simulink model "Demo_DSRC_DNPW_cs"  (Simulink 7.6)
settings: Solver=ode5  SolverMode=SingleTasking  StartTime=0.0  StopTime=5  FixedStep=1/20  RelTol=1e-3
PreLoadFcn:
  | check_NUTS_defined;
  | 
  | assignin('base',['model_closed_' bdroot],false);
InitFcn:
  | PreScanExperimentInitFcn(bdroot)
StopFcn:
  | PreScanExperimentStopFcn(bdroot)
undefined symbols (not defined in the file): DiscIntNeverNeededParam, spare_1, spare_10, spare_11, spare_12, spare_13, spare_14, spare_15, spare_16, spare_17, spare_18, spare_19, spare_2, spare_3, spare_4, spare_5, spare_6, spare_7, spare_8, spare_9
libraries: PreScanSimulinkLibrary x29, PreScanUsefulBlocks x11, simulink x9, simulink_extras x2
(part 3 of 6)

== system Demo_DSRC_DNPW_cs/STATE_HMI_Warning_Left ==
  State : Inport  SampleTime=TimeStep
  Acceleration : Subsystem  mask(ToSensorWorld){PortName=Acceleration_HMI_Warning_Left, PortIndex=212, PortWidth=3, TimeStep=1/20}
      mask prompts: PortName "Port Name [-]"; PortIndex "Index [-]"; PortWidth "Port Dimensions [-]"; TimeStep "Upload Period [s]"
      mask help: Sends signal(s) from Simulink to the Sensor World
      mask Help:
      | Sends signal(s) from Simulink to the Sensor World.
      | 
      | - Port Name [-]: specifies the name of the output terminal of the Simulink block.
      | - Index [-]: specifies the start position in the output vector sent to the Sensor World
      | - Port dimensions [-]: specifies the width (number of scalars) of the output port
      | - Upload period [s]: specifies the upload period (in seconds) of the port.
      mask Display: port_label('input', 1, PortName)
  Demux : Demux  Outputs=5
  Position : Subsystem  mask(ToSensorWorld){PortName=Position_HMI_Warning_Left, PortIndex=206, PortWidth=3, TimeStep=1/20}
      mask prompts: PortName "Port Name [-]"; PortIndex "Index [-]"; PortWidth "Port Dimensions [-]"; TimeStep "Upload Period [s]"
      mask help: Sends signal(s) from Simulink to the Sensor World
      mask Help:
      | Sends signal(s) from Simulink to the Sensor World.
      | 
      | - Port Name [-]: specifies the name of the output terminal of the Simulink block.
      | - Index [-]: specifies the start position in the output vector sent to the Sensor World
      | - Port dimensions [-]: specifies the width (number of scalars) of the output port
      | - Upload period [s]: specifies the upload period (in seconds) of the port.
      mask Display: port_label('input', 1, PortName)
  RPY : Subsystem  mask(ToSensorWorld){PortName=RPY_HMI_Warning_Left, PortIndex=215, PortWidth=3, TimeStep=1/20}
      mask prompts: PortName "Port Name [-]"; PortIndex "Index [-]"; PortWidth "Port Dimensions [-]"; TimeStep "Upload Period [s]"
      mask help: Sends signal(s) from Simulink to the Sensor World
      mask Help:
      | Sends signal(s) from Simulink to the Sensor World.
      | 
      | - Port Name [-]: specifies the name of the output terminal of the Simulink block.
      | - Index [-]: specifies the start position in the output vector sent to the Sensor World
      | - Port dimensions [-]: specifies the width (number of scalars) of the output port
      | - Upload period [s]: specifies the upload period (in seconds) of the port.
      mask Display: port_label('input', 1, PortName)
  Velocity : Subsystem  mask(ToSensorWorld){PortName=Velocity_HMI_Warning_Left, PortIndex=209, PortWidth=3, TimeStep=1/20}
      mask prompts: PortName "Port Name [-]"; PortIndex "Index [-]"; PortWidth "Port Dimensions [-]"; TimeStep "Upload Period [s]"
      mask help: Sends signal(s) from Simulink to the Sensor World
      mask Help:
      | Sends signal(s) from Simulink to the Sensor World.
      | 
      | - Port Name [-]: specifies the name of the output terminal of the Simulink block.
      | - Index [-]: specifies the start position in the output vector sent to the Sensor World
      | - Port dimensions [-]: specifies the width (number of scalars) of the output port
      | - Upload period [s]: specifies the upload period (in seconds) of the port.
      mask Display: port_label('input', 1, PortName)
  iniBODYAngles wrtVEH [rad] : Constant  Value=[Roll0 Pitch0 0]  SampleTime=TimeStep
  iniVEHAngles wrtGLOB [rad] : Constant  Value=[0 0 Yaw0]  SampleTime=TimeStep
  iniVEHposition wrtGLOB [m] : Constant  Value=[x0 y0 z0]  SampleTime=TimeStep
  state2FullState : PreScanSimulinkLibrary/state2FullState  SystemSampleTime=-1
  velRPY : Subsystem  mask(ToSensorWorld){PortName=velRPY_HMI_Warning_Left, PortIndex=218, PortWidth=3, TimeStep=1/20}
      mask prompts: PortName "Port Name [-]"; PortIndex "Index [-]"; PortWidth "Port Dimensions [-]"; TimeStep "Upload Period [s]"
      mask help: Sends signal(s) from Simulink to the Sensor World
      mask Help:
      | Sends signal(s) from Simulink to the Sensor World.
      | 
      | - Port Name [-]: specifies the name of the output terminal of the Simulink block.
      | - Index [-]: specifies the start position in the output vector sent to the Sensor World
      | - Port dimensions [-]: specifies the width (number of scalars) of the output port
      | - Upload period [s]: specifies the upload period (in seconds) of the port.
      mask Display: port_label('input', 1, PortName)
  wires:
  Demux/5 -> velRPY/1(Y)
  Demux/4 -> RPY/1(Y)
  Demux/3 -> Acceleration/1(Y)
  Demux/2 -> Velocity/1(Y)
  Demux/1 -> Position/1(Y)
  State/1 -> state2FullState/1
  state2FullState/1 -> Demux/1
  iniVEHposition wrtGLOB [m]/1 -> state2FullState/2
  iniBODYAngles wrtVEH [rad]/1 -> state2FullState/3
  iniVEHAngles wrtGLOB [rad]/1 -> state2FullState/4

== system Demo_DSRC_DNPW_cs/STATE_HMI_Warning_Right ==
  State : Inport  SampleTime=TimeStep
  Acceleration : Subsystem  mask(ToSensorWorld){PortName=Acceleration_HMI_Warning_Right, PortIndex=227, PortWidth=3, TimeStep=1/20}
      mask prompts: PortName "Port Name [-]"; PortIndex "Index [-]"; PortWidth "Port Dimensions [-]"; TimeStep "Upload Period [s]"
      mask help: Sends signal(s) from Simulink to the Sensor World
      mask Help:
      | Sends signal(s) from Simulink to the Sensor World.
      | 
      | - Port Name [-]: specifies the name of the output terminal of the Simulink block.
      | - Index [-]: specifies the start position in the output vector sent to the Sensor World
      | - Port dimensions [-]: specifies the width (number of scalars) of the output port
      | - Upload period [s]: specifies the upload period (in seconds) of the port.
      mask Display: port_label('input', 1, PortName)
  Demux : Demux  Outputs=5
  Position : Subsystem  mask(ToSensorWorld){PortName=Position_HMI_Warning_Right, PortIndex=221, PortWidth=3, TimeStep=1/20}
      mask prompts: PortName "Port Name [-]"; PortIndex "Index [-]"; PortWidth "Port Dimensions [-]"; TimeStep "Upload Period [s]"
      mask help: Sends signal(s) from Simulink to the Sensor World
      mask Help:
      | Sends signal(s) from Simulink to the Sensor World.
      | 
      | - Port Name [-]: specifies the name of the output terminal of the Simulink block.
      | - Index [-]: specifies the start position in the output vector sent to the Sensor World
      | - Port dimensions [-]: specifies the width (number of scalars) of the output port
      | - Upload period [s]: specifies the upload period (in seconds) of the port.
      mask Display: port_label('input', 1, PortName)
  RPY : Subsystem  mask(ToSensorWorld){PortName=RPY_HMI_Warning_Right, PortIndex=230, PortWidth=3, TimeStep=1/20}
      mask prompts: PortName "Port Name [-]"; PortIndex "Index [-]"; PortWidth "Port Dimensions [-]"; TimeStep "Upload Period [s]"
      mask help: Sends signal(s) from Simulink to the Sensor World
      mask Help:
      | Sends signal(s) from Simulink to the Sensor World.
      | 
      | - Port Name [-]: specifies the name of the output terminal of the Simulink block.
      | - Index [-]: specifies the start position in the output vector sent to the Sensor World
      | - Port dimensions [-]: specifies the width (number of scalars) of the output port
      | - Upload period [s]: specifies the upload period (in seconds) of the port.
      mask Display: port_label('input', 1, PortName)
  Velocity : Subsystem  mask(ToSensorWorld){PortName=Velocity_HMI_Warning_Right, PortIndex=224, PortWidth=3, TimeStep=1/20}
      mask prompts: PortName "Port Name [-]"; PortIndex "Index [-]"; PortWidth "Port Dimensions [-]"; TimeStep "Upload Period [s]"
      mask help: Sends signal(s) from Simulink to the Sensor World
      mask Help:
      | Sends signal(s) from Simulink to the Sensor World.
      | 
      | - Port Name [-]: specifies the name of the output terminal of the Simulink block.
      | - Index [-]: specifies the start position in the output vector sent to the Sensor World
      | - Port dimensions [-]: specifies the width (number of scalars) of the output port
      | - Upload period [s]: specifies the upload period (in seconds) of the port.
      mask Display: port_label('input', 1, PortName)
  iniBODYAngles wrtVEH [rad] : Constant  Value=[Roll0 Pitch0 0]  SampleTime=TimeStep
  iniVEHAngles wrtGLOB [rad] : Constant  Value=[0 0 Yaw0]  SampleTime=TimeStep
  iniVEHposition wrtGLOB [m] : Constant  Value=[x0 y0 z0]  SampleTime=TimeStep
  state2FullState : PreScanSimulinkLibrary/state2FullState  SystemSampleTime=-1
  velRPY : Subsystem  mask(ToSensorWorld){PortName=velRPY_HMI_Warning_Right, PortIndex=233, PortWidth=3, TimeStep=1/20}
      mask prompts: PortName "Port Name [-]"; PortIndex "Index [-]"; PortWidth "Port Dimensions [-]"; TimeStep "Upload Period [s]"
      mask help: Sends signal(s) from Simulink to the Sensor World
      mask Help:
      | Sends signal(s) from Simulink to the Sensor World.
      | 
      | - Port Name [-]: specifies the name of the output terminal of the Simulink block.
      | - Index [-]: specifies the start position in the output vector sent to the Sensor World
      | - Port dimensions [-]: specifies the width (number of scalars) of the output port
      | - Upload period [s]: specifies the upload period (in seconds) of the port.
      mask Display: port_label('input', 1, PortName)
  wires:
  Demux/5 -> velRPY/1(Y)
  Demux/4 -> RPY/1(Y)
  Demux/3 -> Acceleration/1(Y)
  Demux/2 -> Velocity/1(Y)
  Demux/1 -> Position/1(Y)
  State/1 -> state2FullState/1
  state2FullState/1 -> Demux/1
  iniVEHposition wrtGLOB [m]/1 -> state2FullState/2
  iniBODYAngles wrtVEH [rad]/1 -> state2FullState/3
  iniVEHAngles wrtGLOB [rad]/1 -> state2FullState/4

== system Demo_DSRC_DNPW_cs/STATE_Nissan_Cabstar_1 ==
  State : Inport  SampleTime=TimeStep
  Acceleration : Subsystem  mask(ToSensorWorld){PortName=Acceleration_Nissan_Cabstar_1, PortIndex=6, PortWidth=3, TimeStep=1/20}
      mask prompts: PortName "Port Name [-]"; PortIndex "Index [-]"; PortWidth "Port Dimensions [-]"; TimeStep "Upload Period [s]"
      mask help: Sends signal(s) from Simulink to the Sensor World
      mask Help:
      | Sends signal(s) from Simulink to the Sensor World.
      | 
      | - Port Name [-]: specifies the name of the output terminal of the Simulink block.
      | - Index [-]: specifies the start position in the output vector sent to the Sensor World
      | - Port dimensions [-]: specifies the width (number of scalars) of the output port
      | - Upload period [s]: specifies the upload period (in seconds) of the port.
      mask Display: port_label('input', 1, PortName)
  Demux : Demux  Outputs=5
  Position : Subsystem  mask(ToSensorWorld){PortName=Position_Nissan_Cabstar_1, PortIndex=0, PortWidth=3, TimeStep=1/20}
      mask prompts: PortName "Port Name [-]"; PortIndex "Index [-]"; PortWidth "Port Dimensions [-]"; TimeStep "Upload Period [s]"
      mask help: Sends signal(s) from Simulink to the Sensor World
      mask Help:
      | Sends signal(s) from Simulink to the Sensor World.
      | 
      | - Port Name [-]: specifies the name of the output terminal of the Simulink block.
      | - Index [-]: specifies the start position in the output vector sent to the Sensor World
      | - Port dimensions [-]: specifies the width (number of scalars) of the output port
      | - Upload period [s]: specifies the upload period (in seconds) of the port.
      mask Display: port_label('input', 1, PortName)
  RPY : Subsystem  mask(ToSensorWorld){PortName=RPY_Nissan_Cabstar_1, PortIndex=9, PortWidth=3, TimeStep=1/20}
      mask prompts: PortName "Port Name [-]"; PortIndex "Index [-]"; PortWidth "Port Dimensions [-]"; TimeStep "Upload Period [s]"
      mask help: Sends signal(s) from Simulink to the Sensor World
      mask Help:
      | Sends signal(s) from Simulink to the Sensor World.
      | 
      | - Port Name [-]: specifies the name of the output terminal of the Simulink block.
      | - Index [-]: specifies the start position in the output vector sent to the Sensor World
      | - Port dimensions [-]: specifies the width (number of scalars) of the output port
      | - Upload period [s]: specifies the upload period (in seconds) of the port.
      mask Display: port_label('input', 1, PortName)
  Velocity : Subsystem  mask(ToSensorWorld){PortName=Velocity_Nissan_Cabstar_1, PortIndex=3, PortWidth=3, TimeStep=1/20}
      mask prompts: PortName "Port Name [-]"; PortIndex "Index [-]"; PortWidth "Port Dimensions [-]"; TimeStep "Upload Period [s]"
      mask help: Sends signal(s) from Simulink to the Sensor World
      mask Help:
      | Sends signal(s) from Simulink to the Sensor World.
      | 
      | - Port Name [-]: specifies the name of the output terminal of the Simulink block.
      | - Index [-]: specifies the start position in the output vector sent to the Sensor World
      | - Port dimensions [-]: specifies the width (number of scalars) of the output port
      | - Upload period [s]: specifies the upload period (in seconds) of the port.
      mask Display: port_label('input', 1, PortName)
  iniBODYAngles wrtVEH [rad] : Constant  Value=[Roll0 Pitch0 0]  SampleTime=TimeStep
  iniVEHAngles wrtGLOB [rad] : Constant  Value=[0 0 Yaw0]  SampleTime=TimeStep
  iniVEHposition wrtGLOB [m] : Constant  Value=[x0 y0 z0]  SampleTime=TimeStep
  state2FullState : PreScanSimulinkLibrary/state2FullState  SystemSampleTime=-1
  velRPY : Subsystem  mask(ToSensorWorld){PortName=velRPY_Nissan_Cabstar_1, PortIndex=12, PortWidth=3, TimeStep=1/20}
      mask prompts: PortName "Port Name [-]"; PortIndex "Index [-]"; PortWidth "Port Dimensions [-]"; TimeStep "Upload Period [s]"
      mask help: Sends signal(s) from Simulink to the Sensor World
      mask Help:
      | Sends signal(s) from Simulink to the Sensor World.
      | 
      | - Port Name [-]: specifies the name of the output terminal of the Simulink block.
      | - Index [-]: specifies the start position in the output vector sent to the Sensor World
      | - Port dimensions [-]: specifies the width (number of scalars) of the output port
      | - Upload period [s]: specifies the upload period (in seconds) of the port.
      mask Display: port_label('input', 1, PortName)
  wires:
  Demux/5 -> velRPY/1(Y)
  Demux/4 -> RPY/1(Y)
  Demux/3 -> Acceleration/1(Y)
  Demux/2 -> Velocity/1(Y)
  Demux/1 -> Position/1(Y)
  State/1 -> state2FullState/1
  state2FullState/1 -> Demux/1
  iniVEHposition wrtGLOB [m]/1 -> state2FullState/2
  iniBODYAngles wrtVEH [rad]/1 -> state2FullState/3
  iniVEHAngles wrtGLOB [rad]/1 -> state2FullState/4

== system Demo_DSRC_DNPW_cs/STATE_Toyota_Yaris_1 ==
  State : Inport  SampleTime=TimeStep
  Acceleration : Subsystem  mask(ToSensorWorld){PortName=Acceleration_Toyota_Yaris_1, PortIndex=110, PortWidth=3, TimeStep=1/20}
      mask prompts: PortName "Port Name [-]"; PortIndex "Index [-]"; PortWidth "Port Dimensions [-]"; TimeStep "Upload Period [s]"
      mask help: Sends signal(s) from Simulink to the Sensor World
      mask Help:
      | Sends signal(s) from Simulink to the Sensor World.
      | 
      | - Port Name [-]: specifies the name of the output terminal of the Simulink block.
      | - Index [-]: specifies the start position in the output vector sent to the Sensor World
      | - Port dimensions [-]: specifies the width (number of scalars) of the output port
      | - Upload period [s]: specifies the upload period (in seconds) of the port.
      mask Display: port_label('input', 1, PortName)
  Demux : Demux  Outputs=5
  Position : Subsystem  mask(ToSensorWorld){PortName=Position_Toyota_Yaris_1, PortIndex=104, PortWidth=3, TimeStep=1/20}
      mask prompts: PortName "Port Name [-]"; PortIndex "Index [-]"; PortWidth "Port Dimensions [-]"; TimeStep "Upload Period [s]"
      mask help: Sends signal(s) from Simulink to the Sensor World
      mask Help:
      | Sends signal(s) from Simulink to the Sensor World.
      | 
      | - Port Name [-]: specifies the name of the output terminal of the Simulink block.
      | - Index [-]: specifies the start position in the output vector sent to the Sensor World
      | - Port dimensions [-]: specifies the width (number of scalars) of the output port
      | - Upload period [s]: specifies the upload period (in seconds) of the port.
      mask Display: port_label('input', 1, PortName)
  RPY : Subsystem  mask(ToSensorWorld){PortName=RPY_Toyota_Yaris_1, PortIndex=113, PortWidth=3, TimeStep=1/20}
      mask prompts: PortName "Port Name [-]"; PortIndex "Index [-]"; PortWidth "Port Dimensions [-]"; TimeStep "Upload Period [s]"
      mask help: Sends signal(s) from Simulink to the Sensor World
      mask Help:
      | Sends signal(s) from Simulink to the Sensor World.
      | 
      | - Port Name [-]: specifies the name of the output terminal of the Simulink block.
      | - Index [-]: specifies the start position in the output vector sent to the Sensor World
      | - Port dimensions [-]: specifies the width (number of scalars) of the output port
      | - Upload period [s]: specifies the upload period (in seconds) of the port.
      mask Display: port_label('input', 1, PortName)
  Velocity : Subsystem  mask(ToSensorWorld){PortName=Velocity_Toyota_Yaris_1, PortIndex=107, PortWidth=3, TimeStep=1/20}
      mask prompts: PortName "Port Name [-]"; PortIndex "Index [-]"; PortWidth "Port Dimensions [-]"; TimeStep "Upload Period [s]"
      mask help: Sends signal(s) from Simulink to the Sensor World
      mask Help:
      | Sends signal(s) from Simulink to the Sensor World.
      | 
      | - Port Name [-]: specifies the name of the output terminal of the Simulink block.
      | - Index [-]: specifies the start position in the output vector sent to the Sensor World
      | - Port dimensions [-]: specifies the width (number of scalars) of the output port
      | - Upload period [s]: specifies the upload period (in seconds) of the port.
      mask Display: port_label('input', 1, PortName)
  iniBODYAngles wrtVEH [rad] : Constant  Value=[Roll0 Pitch0 0]  SampleTime=TimeStep
  iniVEHAngles wrtGLOB [rad] : Constant  Value=[0 0 Yaw0]  SampleTime=TimeStep
  iniVEHposition wrtGLOB [m] : Constant  Value=[x0 y0 z0]  SampleTime=TimeStep
  state2FullState : PreScanSimulinkLibrary/state2FullState  SystemSampleTime=-1
  velRPY : Subsystem  mask(ToSensorWorld){PortName=velRPY_Toyota_Yaris_1, PortIndex=116, PortWidth=3, TimeStep=1/20}
      mask prompts: PortName "Port Name [-]"; PortIndex "Index [-]"; PortWidth "Port Dimensions [-]"; TimeStep "Upload Period [s]"
      mask help: Sends signal(s) from Simulink to the Sensor World
      mask Help:
      | Sends signal(s) from Simulink to the Sensor World.
      | 
      | - Port Name [-]: specifies the name of the output terminal of the Simulink block.
      | - Index [-]: specifies the start position in the output vector sent to the Sensor World
      | - Port dimensions [-]: specifies the width (number of scalars) of the output port
      | - Upload period [s]: specifies the upload period (in seconds) of the port.
      mask Display: port_label('input', 1, PortName)
  wires:
  Demux/5 -> velRPY/1(Y)
  Demux/4 -> RPY/1(Y)
  Demux/3 -> Acceleration/1(Y)
  Demux/2 -> Velocity/1(Y)
  Demux/1 -> Position/1(Y)
  State/1 -> state2FullState/1
  state2FullState/1 -> Demux/1
  iniVEHposition wrtGLOB [m]/1 -> state2FullState/2
  iniBODYAngles wrtVEH [rad]/1 -> state2FullState/3
  iniVEHAngles wrtGLOB [rad]/1 -> state2FullState/4

== system Demo_DSRC_DNPW_cs/Scope Collision Detections ==
  In1 : Inport
  Collision Detections : Scope  NumInputPorts=5
      settings: YMin=0~0~0~0~0  YMax=10~10~10~10~10  SaveName=ScopeData2
  Demux2 : Demux  Outputs=5
  wires:
  Demux2/1 -> Collision Detections/1
  Demux2/2 -> Collision Detections/2
  Demux2/3 -> Collision Detections/3
  Demux2/4 -> Collision Detections/4
  Demux2/5 -> Collision Detections/5
  In1/1 -> Demux2/1

== system Demo_DSRC_DNPW_cs/Scope Collision IDs ==
  In1 : Inport
  Collision IDs : Scope  NumInputPorts=5
      settings: YMin=0~0~0~0~0  YMax=10~10~10~10~10  SaveName=ScopeData2
  Demux2 : Demux  Outputs=5
  wires:
  In1/1 -> Demux2/1
  Demux2/5 -> Collision IDs/5
  Demux2/4 -> Collision IDs/4
  Demux2/3 -> Collision IDs/3
  Demux2/2 -> Collision IDs/2
  Demux2/1 -> Collision IDs/1

== system Demo_DSRC_DNPW_cs/SetActuators ==
  Bus Creator : BusCreator  Inputs=1
  Data Store Read : DataStoreRead  DataStoreName=SimCoreActuators  SampleTime=TimeStep
  SendActuators : M-S-Function  FunctionName=SendActuatorsBlock  Parameters=TimeStep NrOfActuators
  dummy : Outport
  tag scope: SimCoreInfo=global
  wires:
  Bus Creator/1 -> [SimCoreInfo]  "SimCore"
  SendActuators/2 -> Bus Creator/1  "ComputationTime[s]"
  SendActuators/1 -> dummy/1
  Data Store Read/1 -> SendActuators/1

== system Demo_DSRC_DNPW_cs/SimCoreInfo ==
  Bus Selector : BusSelector  OutputSignals=ComputationTime[s]
  Time : Scope
      settings: TimeRange=10  YMin=0  YMax=0.5  SaveName=ComputationTime
  wires:
  Bus Selector/1 -> Time/1  "<ComputationTime[s]>"
  [SimCoreInfo] -> Bus Selector/1

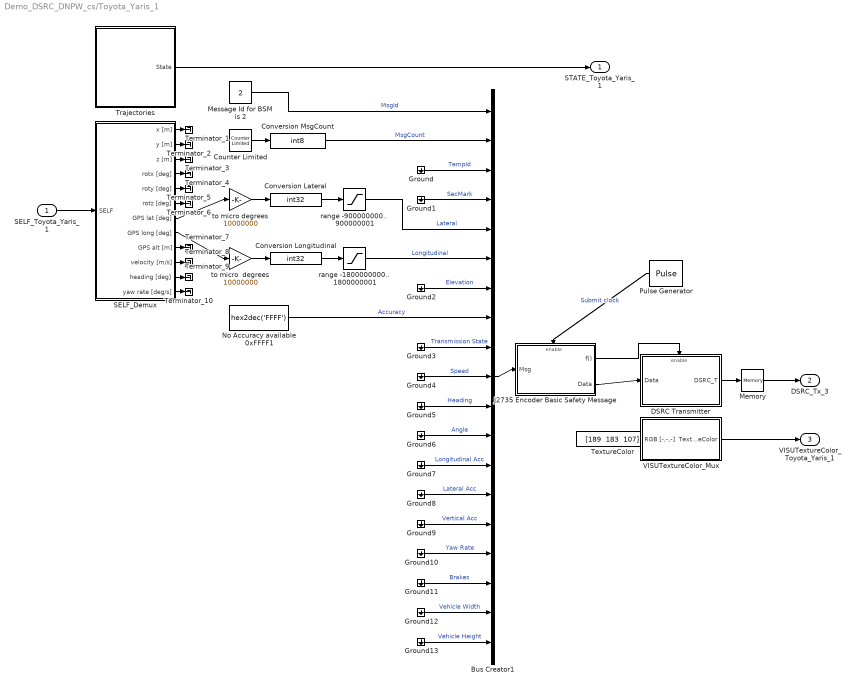
== system Demo_DSRC_DNPW_cs/Toyota_Yaris_1 ==
  SELF_Toyota_Yaris_1 : Inport  Tag=SELFInport
  Bus Creator1 : BusCreator  Inputs=19
  Conversion Lateral : DataTypeConversion  OutDataTypeStr=int32
  Conversion Longitudinal : DataTypeConversion  OutDataTypeStr=int32
  Conversion MsgCount : DataTypeConversion  OutDataTypeStr=int8
  Counter Limited : simulink/Sources/Counter Limited  SystemSampleTime=-1  uplimit=127  tsamp=-1
  DSRC Transmitter : Subsystem  Tag=DSRC_Transmitter
  Ground{,1..13} (14 alike) : Ground
  J2735 Encoder Basic Safety Message : Subsystem  Tag=J2735_Encoder_Basic_Safety_Message
  Memory : Memory
  Message Id for BSM is 2 : Constant  Value=2  OutDataTypeStr=int8
  No Accuracy available 0xFFFF1 : Constant  Value=hex2dec('FFFF')  OutDataTypeStr=int32
  Pulse Generator : DiscretePulseGenerator  Period=1  SampleTime=1/20
  SELF_Demux : Subsystem  Tag=DemuxSELF
      settings: DeleteFcn=PreScanBlockDeleteFcn;
      mask Type: PreScan Demux Block:
      mask Display:
      | port_label('output',1,'x [m]')
      | port_label('output',2,'y [m]')
      | port_label('output',3,'z [m]','texmode','on')
      | port_label('output',4,'Rotx [deg]','texmode','on')
      | port_label('output',5,'Roty [deg]','texmode','on')
      | port_label('output',6,'Rotz [deg]','texmode','on')
      | port_label('output',7,'GPS lat [deg]','texmode','on')
      | port_label('output',8,'GPS long [deg]','texmode','on')
      | port_label('output',9,'GPS alt [m]','texmode','on')
      | port_label('output',10,'Velocity [m/s]')
      | port_label('output',11,'Heading [deg]')
      | port_label('output',12,'Yaw rate [deg/s]')
  Terminator_{1..10} (10 alike) : Terminator
  TextureColor : Constant  Tag=TextureColor  Value="[189  183  107]"
  Trajectories : Subsystem  Tag=Trajectories
      settings: DeleteFcn=PreScanBlockDeleteFcn;
      mask Type: PreScan Source Block: Trajectories
      mask Description:
      | The Trajectory block contains the trajectories defined in the PreScan Experiment Editor. The output of the trajectory block is the (vehicle) State.
      | 
      | For more information, please click Help.
      mask Help: eval('openHelp(312)')
      mask Display: image(imread('Trajectory.png'));
  VISUTextureColor_Mux : Subsystem  Tag=MuxSteer
      settings: DeleteFcn=PreScanBlockDeleteFcn;
      mask Type: PreScan Mux Block:
  range -1800000000..  1800000001 : Saturate  UpperLimit=1800000001  LowerLimit=-1800000000  OutDataTypeStr=int32
  range -900000000..  900000001 : Saturate  UpperLimit=900000001  LowerLimit=-900000000  OutDataTypeStr=int32
  to micro degrees : Gain  Gain=10000000
  to micro  degrees : Gain  Gain=10000000
  STATE_Toyota_Yaris_1 : Outport  Tag=StateOutport
  DSRC_Tx_3 : Outport  Tag=DSRC_TOutport  Port=2
  VISUTextureColor_Toyota_Yaris_1 : Outport  Tag=VisuTextureColorOutport  Port=3  SampleTime=1/20
  wires:
  Message Id for BSM is 2/1 -> Bus Creator1/1  "MsgId"
  Counter Limited/1 -> Conversion MsgCount/1
  to micro  degrees/1 -> Conversion Longitudinal/1
  Conversion Longitudinal/1 -> range -1800000000..  1800000001/1
  Conversion Lateral/1 -> range -900000000..  900000001/1
  to micro degrees/1 -> Conversion Lateral/1
  No Accuracy available 0xFFFF1/1 -> Bus Creator1/8  "Accuracy"
  Ground13/1 -> Bus Creator1/19  "Vehicle Height"
  Ground12/1 -> Bus Creator1/18  "Vehicle Width"
  Ground11/1 -> Bus Creator1/17  "Brakes"
  Ground10/1 -> Bus Creator1/16  "Yaw Rate"
  Ground9/1 -> Bus Creator1/15  "Vertical Acc"
  Ground8/1 -> Bus Creator1/14  "Lateral Acc"
  Ground7/1 -> Bus Creator1/13  "Longitudinal Acc"
  Ground6/1 -> Bus Creator1/12  "Angle"
  Ground2/1 -> Bus Creator1/7  "Elevation"
  Ground1/1 -> Bus Creator1/4  "SecMark"
  Ground/1 -> Bus Creator1/3  "TempId"
  Conversion MsgCount/1 -> Bus Creator1/2  "MsgCount"
  range -900000000..  900000001/1 -> Bus Creator1/5  "Lateral"
  range -1800000000..  1800000001/1 -> Bus Creator1/6  "Longitudinal"
  Ground5/1 -> Bus Creator1/11  "Heading"
  Ground4/1 -> Bus Creator1/10  "Speed"
  Ground3/1 -> Bus Creator1/9  "Transmission State"
  SELF_Toyota_Yaris_1/1 -> SELF_Demux/1(SELF)
  J2735 Encoder Basic Safety Message/1(f()) -> DSRC Transmitter/Enable
  J2735 Encoder Basic Safety Message/2(Data) -> DSRC Transmitter/1(Data)
  DSRC Transmitter/1(DSRC_T) -> Memory/1
  VISUTextureColor_Mux/1(TextureColor) -> VISUTextureColor_Toyota_Yaris_1/1
  TextureColor/1 -> VISUTextureColor_Mux/1(RGB [-,-,-])
  Trajectories/1(State) -> STATE_Toyota_Yaris_1/1
  Pulse Generator/1 -> J2735 Encoder Basic Safety Message/Enable  "Submit clock"
  SELF_Demux/7(GPS lat [deg]) -> to micro degrees/1
  SELF_Demux/8(GPS long [deg]) -> to micro  degrees/1
  Bus Creator1/1 -> J2735 Encoder Basic Safety Message/1(Msg)
  Memory/1 -> DSRC_Tx_3/1
  SELF_Demux/1(x [m]) -> Terminator_1/1
  SELF_Demux/2(y [m]) -> Terminator_2/1
  SELF_Demux/3(z [m]) -> Terminator_3/1
  SELF_Demux/4(rotx [deg]) -> Terminator_4/1
  SELF_Demux/5(roty [deg]) -> Terminator_5/1
  SELF_Demux/6(rotz [deg]) -> Terminator_6/1
  SELF_Demux/9(GPS alt [m]) -> Terminator_7/1
  SELF_Demux/10(velocity [m/s]) -> Terminator_8/1
  SELF_Demux/11(heading [deg]) -> Terminator_9/1
  SELF_Demux/12(yaw rate [deg/s]) -> Terminator_10/1

== system Demo_DSRC_DNPW_cs/VISUSteer_BMW_X5_1 ==
  Steer : Inport
  Demux3 : Demux  Outputs=[1 1]
  Saturation : Saturate  UpperLimit=30  LowerLimit=-5
  Saturation1 : Saturate  UpperLimit=720  LowerLimit=-720
  conv_SteeringColumn : Subsystem
  conv_SteeringWheel : Subsystem
  visu_SteeringColumn : Subsystem  mask(ToSensorWorld){PortName=visu_SteeringColumn_0, PortIndex=100, PortWidth=4, TimeStep=1/20}
      mask prompts: PortName "Port Name [-]"; PortIndex "Index [-]"; PortWidth "Port Dimensions [-]"; TimeStep "Upload Period [s]"
      mask help: Sends signal(s) from Simulink to the Sensor World
      mask Help:
      | Sends signal(s) from Simulink to the Sensor World.
      | 
      | - Port Name [-]: specifies the name of the output terminal of the Simulink block.
      | - Index [-]: specifies the start position in the output vector sent to the Sensor World
      | - Port dimensions [-]: specifies the width (number of scalars) of the output port
      | - Upload period [s]: specifies the upload period (in seconds) of the port.
      mask Display: port_label('input', 1, PortName)
  visu_SteeringWheel : Subsystem  mask(ToSensorWorld){PortName=visu_SteeringWheel_0, PortIndex=96, PortWidth=4, TimeStep=1/20}
      mask prompts: PortName "Port Name [-]"; PortIndex "Index [-]"; PortWidth "Port Dimensions [-]"; TimeStep "Upload Period [s]"
      mask help: Sends signal(s) from Simulink to the Sensor World
      mask Help:
      | Sends signal(s) from Simulink to the Sensor World.
      | 
      | - Port Name [-]: specifies the name of the output terminal of the Simulink block.
      | - Index [-]: specifies the start position in the output vector sent to the Sensor World
      | - Port dimensions [-]: specifies the width (number of scalars) of the output port
      | - Upload period [s]: specifies the upload period (in seconds) of the port.
      mask Display: port_label('input', 1, PortName)
  wires:
  conv_SteeringColumn/1(QuaternionVisu [rad]) -> visu_SteeringColumn/1(Y)
  conv_SteeringWheel/1(QuaternionVisu [rad]) -> visu_SteeringWheel/1(Y)
  Demux3/2 -> Saturation/1
  Demux3/1 -> Saturation1/1
  Saturation1/1 -> conv_SteeringWheel/1(angle [deg])
  Saturation/1 -> conv_SteeringColumn/1(angle [deg])
  Steer/1 -> Demux3/1

== system Demo_DSRC_DNPW_cs/VISUTextureColor_Fiat_Bravo_1 ==
  TextureColor : Inport
  visu_TextureColor : Subsystem  mask(ToSensorWorld){PortName=visu_TextureColor_0, PortIndex=78, PortWidth=3, TimeStep=1/20}
      mask prompts: PortName "Port Name [-]"; PortIndex "Index [-]"; PortWidth "Port Dimensions [-]"; TimeStep "Upload Period [s]"
      mask help: Sends signal(s) from Simulink to the Sensor World
      mask Help:
      | Sends signal(s) from Simulink to the Sensor World.
      | 
      | - Port Name [-]: specifies the name of the output terminal of the Simulink block.
      | - Index [-]: specifies the start position in the output vector sent to the Sensor World
      | - Port dimensions [-]: specifies the width (number of scalars) of the output port
      | - Upload period [s]: specifies the upload period (in seconds) of the port.
      mask Display: port_label('input', 1, PortName)
  wires:
  TextureColor/1 -> visu_TextureColor/1(Y)

== system Demo_DSRC_DNPW_cs/VISUTextureColor_Toyota_Yaris_1 ==
  TextureColor : Inport
  visu_TextureColor : Subsystem  mask(ToSensorWorld){PortName=visu_TextureColor_0, PortIndex=143, PortWidth=3, TimeStep=1/20}
      mask prompts: PortName "Port Name [-]"; PortIndex "Index [-]"; PortWidth "Port Dimensions [-]"; TimeStep "Upload Period [s]"
      mask help: Sends signal(s) from Simulink to the Sensor World
      mask Help:
      | Sends signal(s) from Simulink to the Sensor World.
      | 
      | - Port Name [-]: specifies the name of the output terminal of the Simulink block.
      | - Index [-]: specifies the start position in the output vector sent to the Sensor World
      | - Port dimensions [-]: specifies the width (number of scalars) of the output port
      | - Upload period [s]: specifies the upload period (in seconds) of the port.
      mask Display: port_label('input', 1, PortName)
  wires:
  TextureColor/1 -> visu_TextureColor/1(Y)

== system Demo_DSRC_DNPW_cs/BMW_X5_1/DNPW ==
  Range : Inport
  Theta : Inport  Port=2
  Yaw Rate : Inport  Port=3
  Abs : Abs
  Forward Zone : Subsystem
  Left Zone : Subsystem
  Logical Operator{,1..6} (7 alike) : Logic  AllPortsSameDT=off  OutDataTypeStr=boolean
  Relational Operator : RelationalOperator  Operator=<  OutDataTypeStr=boolean
  Relational Operator1 : RelationalOperator  OutDataTypeStr=boolean
  Relational Operator2 : RelationalOperator  Operator=<=  OutDataTypeStr=boolean
  Right Zone : Subsystem
  Signal Delay : Subsystem
  Signal Delay1 : Subsystem
  Signal Delay2 : Subsystem
  Unary Minus : UnaryMinus
  Left Reminding : Outport
  Right Reminding : Outport  Port=2
  Left Warning : Outport  Port=3
  Right Warning : Outport  Port=4
  wires:
  Range/1 -> Left Zone/1(Range), Right Zone/1(Range), Forward Zone/1(Range)
  Theta/1 -> Left Zone/2(Theta), Right Zone/2(Theta), Forward Zone/2(Theta)
  Yaw Rate/1 -> Abs/1, Relational Operator1/1, Relational Operator2/1
  Forward Zone/1(Out1) -> Logical Operator/1
  Logical Operator/1 -> Signal Delay/1(In1)
  Relational Operator/1 -> Logical Operator/2, Logical Operator1/2, Logical Operator2/2
  Left Zone/1(Out1) -> Logical Operator1/1
  Logical Operator1/1 -> Signal Delay1/1(In1)
  Right Zone/1(Out1) -> Logical Operator2/1
  Logical Operator2/1 -> Signal Delay2/1(In1)
  Signal Delay1/1(Out1) -> Logical Operator3/2
  Signal Delay/1(Out1) -> Logical Operator3/1, Logical Operator4/1
  Signal Delay2/1(Out1) -> Logical Operator4/2
  Logical Operator3/1 -> Left Reminding/1, Logical Operator5/1
  Logical Operator4/1 -> Right Reminding/1, Logical Operator6/1
  Relational Operator1/1 -> Logical Operator5/2
  Relational Operator2/1 -> Logical Operator6/2
  Logical Operator5/1 -> Left Warning/1
  Logical Operator6/1 -> Right Warning/1
  Abs/1 -> Relational Operator/1
  [SEYawrate] -> Relational Operator/2
  [SWYawrate] -> Relational Operator1/2
  [SWYawrate] -> Unary Minus/1
  Unary Minus/1 -> Relational Operator2/2

== system Demo_DSRC_DNPW_cs/BMW_X5_1/DSRC Receiver ==
  In1 : Inport
  Always Enabled : Constant
  Bus Selector : BusSelector  OutputSignals=spare_1,spare_2,spare_3,spare_4,spare_5,spare_6,spare_7,spare_8,spare_9,spare_10,spare_11,spare_12,spare_13,spare_14,spare_15,spare_16,spare_17,spare_18,spare_19  OutputAsBus=on
  Bus to Vector : BusToVector
  DSRC_Rx_Demux : Subsystem  Tag=DemuxDSRCR
      settings: DeleteFcn=PreScanBlockDeleteFcn;
      mask Type: PreScan Demux Block:
      mask Display:
      | port_label('output', 1, 'Vehicle_ID')
      | port_label('output', 2, 'GPS Pos Lat [deg]')
      | port_label('output', 3, 'GPS Pos Long [deg]')
      | port_label('output', 4, 'GPS Pos Alt [m]')
      | port_label('output', 5, 'Velocity [m/s]')
      | port_label('output', 6, 'Acceleration [m/s2]')
      | port_label('output', 7, 'Heading [deg]')
      | port_label('output', 8, 'Warning signal ID')
      | port_label('output', 9, 'Maneuvre ID')
      | port_label('output', 10, 'Vehicle Type')
      | port_label('output', 11, 'Braking Capacity')
      | port_label('output', 12, 'Vehicle Size')
      | port_label('output', 13, 'Spare')
  Terminator_{2..13} (12 alike) : Terminator
  f() : Outport
  Data : Outport  Port=2
  wires:
  Bus to Vector/1 -> Data/1
  Bus Selector/1 -> Bus to Vector/1
  DSRC_Rx_Demux/13(spare) -> Bus Selector/1  "L7"
  Always Enabled/1 -> f()/1  "Enable"
  In1/1 -> DSRC_Rx_Demux/1(AntennaR)
  DSRC_Rx_Demux/12(vehicle_size) -> Terminator_13/1
  DSRC_Rx_Demux/11(brakingcapacity) -> Terminator_12/1
  DSRC_Rx_Demux/10(vehicle_type) -> Terminator_11/1
  DSRC_Rx_Demux/9(maneuvre_id) -> Terminator_10/1
  DSRC_Rx_Demux/8(warning_signal_id) -> Terminator_9/1
  DSRC_Rx_Demux/7(Heading [deg]) -> Terminator_8/1
  DSRC_Rx_Demux/6(Acceleration_[m/s2]) -> Terminator_7/1
  DSRC_Rx_Demux/5(Velocity_[m/s]) -> Terminator_6/1
  DSRC_Rx_Demux/4(GPS_pos_alt_[m]) -> Terminator_5/1
  DSRC_Rx_Demux/3(GPS_pos_long_[deg]) -> Terminator_4/1
  DSRC_Rx_Demux/2(GPS_pos_lat_[deg]) -> Terminator_3/1
  DSRC_Rx_Demux/1(Vehicle_ID) -> Terminator_2/1

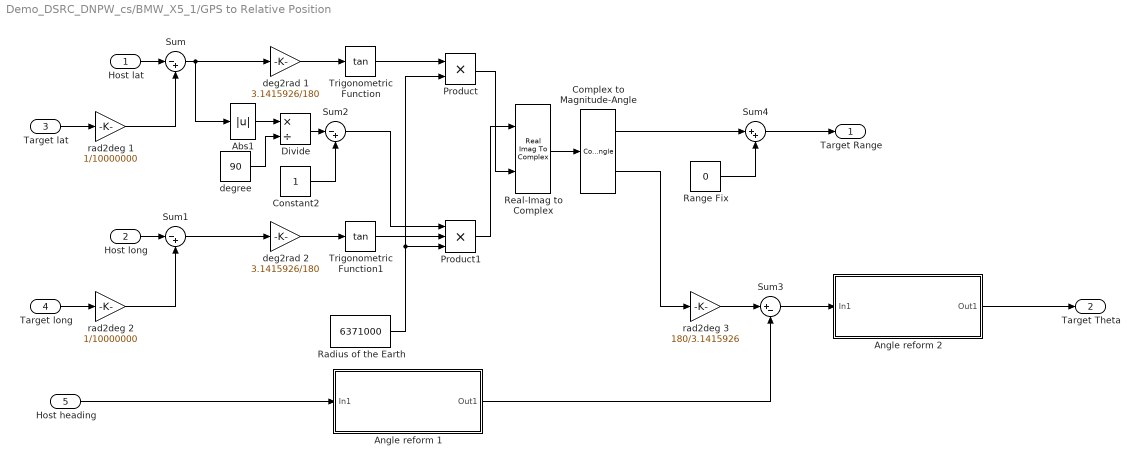
== system Demo_DSRC_DNPW_cs/BMW_X5_1/GPS to Relative Position ==
  Host lat : Inport
  Host long : Inport  Port=2
  Target lat : Inport  Port=3
  Target long : Inport  Port=4
  Host heading : Inport  Port=5
  Abs1 : Abs
  "Angle reform 1 " : Subsystem
  Angle reform 2 : Subsystem
  Complex to Magnitude-Angle : ComplexToMagnitudeAngle
  Constant2 : Constant
  Divide : Product  Inputs=*/
  Product : Product  RndMeth=Zero
  Product1 : Product  Inputs=3  RndMeth=Zero
  Radius of the Earth : Constant  Value=6371000
  Range Fix : Constant  Value=0
  Real-Imag to Complex : RealImagToComplex
  Sum : Sum  Inputs=|-+
  Sum1 : Sum  Inputs=|-+
  Sum2 : Sum  Inputs=|-+
  Sum3 : Sum  Inputs=|+-
  Sum4 : Sum  Inputs=|++
  Trigonometric Function : Trigonometry  Operator=tan
  Trigonometric Function1 : Trigonometry  Operator=tan
  deg2rad 1 : Gain  Gain=3.1415926/180
  deg2rad 2 : Gain  Gain=3.1415926/180
  degree : Constant  Value=90
  rad2deg 1 : Gain  Gain=1/10000000  ParamDataTypeStr=double
  rad2deg 2 : Gain  Gain=1/10000000  ParamDataTypeStr=double
  rad2deg 3 : Gain  Gain=180/3.1415926
  Target Range : Outport
  Target Theta : Outport  Port=2
  wires:
  Product/1 -> Real-Imag to Complex/2
  Product1/1 -> Real-Imag to Complex/1
  rad2deg 3/1 -> Sum3/1
  Complex to Magnitude-Angle/2 -> rad2deg 3/1
  Real-Imag to Complex/1 -> Complex to Magnitude-Angle/1
  Abs1/1 -> Divide/1
  Sum2/1 -> Product1/1
  Constant2/1 -> Sum2/2
  Divide/1 -> Sum2/1
  degree/1 -> Divide/2
  Trigonometric Function1/1 -> Product1/2
  Radius of the Earth/1 -> Product/2, Product1/3
  Trigonometric Function/1 -> Product/1
  Sum1/1 -> deg2rad 2/1
  deg2rad 2/1 -> Trigonometric Function1/1
  deg2rad 1/1 -> Trigonometric Function/1
  rad2deg 2/1 -> Sum1/2
  Sum/1 -> deg2rad 1/1, Abs1/1
  rad2deg 1/1 -> Sum/2
  Target lat/1 -> rad2deg 1/1
  Target long/1 -> rad2deg 2/1
  Host lat/1 -> Sum/1
  Host long/1 -> Sum1/1
  Sum3/1 -> Angle reform 2/1(In1)
  Complex to Magnitude-Angle/1 -> Sum4/1
  Sum4/1 -> Target Range/1
  Range Fix/1 -> Sum4/2
  Angle reform 2/1(Out1) -> Target Theta/1
  "Angle reform 1 "/1(Out1) -> Sum3/2
  Host heading/1 -> "Angle reform 1 "/1(In1)

== system Demo_DSRC_DNPW_cs/BMW_X5_1/J2735 Decoder Basic Safety Message ==
  Data : Inport
  Enable : EnablePort  PropagateVarSize=During execution
  Always Enabled : Constant
  Bus Creator : BusCreator  Inputs=19
  Conversion Accuracy : DataTypeConversion  OutDataTypeStr=int32
  Conversion Angle : DataTypeConversion  OutDataTypeStr=int8
  Conversion Brakes : DataTypeConversion  OutDataTypeStr=int16
  Conversion Elevation : DataTypeConversion  OutDataTypeStr=int16
  Conversion Heading : DataTypeConversion  OutDataTypeStr=int16
  Conversion Lateral : DataTypeConversion  OutDataTypeStr=int32
  Conversion Lateral Acc : DataTypeConversion  OutDataTypeStr=int16
  Conversion Longitudinal : DataTypeConversion  OutDataTypeStr=int32
  Conversion Longitudinal Acc : DataTypeConversion  OutDataTypeStr=int16
  Conversion MsgCount : DataTypeConversion  OutDataTypeStr=int8
  Conversion MsgId : DataTypeConversion  OutDataTypeStr=int8
  Conversion SecMark : DataTypeConversion  OutDataTypeStr=uint16
  Conversion Speed : DataTypeConversion  OutDataTypeStr=int16
  Conversion TempId : DataTypeConversion  OutDataTypeStr=int32
  Conversion Transmission State : DataTypeConversion  OutDataTypeStr=int8
  Conversion Vehicle Height : DataTypeConversion  OutDataTypeStr=int16
  Conversion Vehicle Width : DataTypeConversion  OutDataTypeStr=int16
  Conversion Vertical Acc : DataTypeConversion  OutDataTypeStr=int8
  Conversion Yaw Rate : DataTypeConversion  OutDataTypeStr=int16
  Demux : Demux  Outputs=19
  f() : Outport  InitialOutput=[1]
  Msg : Outport  Port=2
  wires:
  Conversion Vehicle Height/1 -> Bus Creator/19  "Vehicle Height"
  Demux/19 -> Conversion Vehicle Height/1
  Conversion Vehicle Width/1 -> Bus Creator/18  "Vehicle Width"
  Conversion Brakes/1 -> Bus Creator/17  "Brakes"
  Demux/18 -> Conversion Vehicle Width/1
  Demux/17 -> Conversion Brakes/1
  Conversion Yaw Rate/1 -> Bus Creator/16  "Yaw Rate"
  Conversion Vertical Acc/1 -> Bus Creator/15  "Vertical Acc"
  Demux/16 -> Conversion Yaw Rate/1
  Demux/15 -> Conversion Vertical Acc/1
  Conversion Lateral Acc/1 -> Bus Creator/14  "Lateral Acc"
  Conversion Longitudinal Acc/1 -> Bus Creator/13  "Longitudinal Acc"
  Demux/14 -> Conversion Lateral Acc/1
  Demux/13 -> Conversion Longitudinal Acc/1
  Conversion Angle/1 -> Bus Creator/12  "Angle"
  Conversion Heading/1 -> Bus Creator/11  "Heading"
  Demux/12 -> Conversion Angle/1
  Demux/11 -> Conversion Heading/1
  Conversion Speed/1 -> Bus Creator/10  "Speed"
  Conversion Transmission State/1 -> Bus Creator/9  "Transmission State"
  Demux/10 -> Conversion Speed/1
  Demux/9 -> Conversion Transmission State/1
  Conversion Accuracy/1 -> Bus Creator/8  "Accuracy"
  Demux/8 -> Conversion Accuracy/1
  Conversion Elevation/1 -> Bus Creator/7  "Elevation"
  Demux/7 -> Conversion Elevation/1
  Conversion Longitudinal/1 -> Bus Creator/6  "Longitudinal"
  Demux/6 -> Conversion Longitudinal/1
  Conversion Lateral/1 -> Bus Creator/5  "Lateral"
  Demux/5 -> Conversion Lateral/1
  Conversion SecMark/1 -> Bus Creator/4  "SecMark"
  Demux/4 -> Conversion SecMark/1
  Conversion TempId/1 -> Bus Creator/3  "TempId"
  Demux/3 -> Conversion TempId/1
  Demux/2 -> Conversion MsgCount/1
  Conversion MsgCount/1 -> Bus Creator/2  "MsgCount"
  Bus Creator/1 -> Msg/1
  Conversion MsgId/1 -> Bus Creator/1  "MsgId"
  Demux/1 -> Conversion MsgId/1
  Data/1 -> Demux/1
  Always Enabled/1 -> f()/1

== system Demo_DSRC_DNPW_cs/BMW_X5_1/SELF_Demux ==
  SELF : Inport
  Demux1 : Demux  Outputs=3
  Demux2 : Demux  Outputs=3
  Demux3 : Demux  Outputs=[3 3 1 1]
  Demux4 : Demux  Outputs=3
  Gain : Gain  Gain=180/pi
  Gain1 : Gain  Gain=180/pi
  Selector : Selector  InputPortWidth=3  IndexOptions=Index vector (dialog)  Indices=[3]  OutputSizes=1
  compas converter : Subsystem
  xyz2GPS : PreScanUsefulBlocks/xyz2GPS  CoordinateCount=1  GPS_base=[0.000000 0.000000 0.000]
  x [m] : Outport
  y [m] : Outport  Port=2
  z [m] : Outport  Port=3
  rotx [deg] : Outport  Port=4
  roty [deg] : Outport  Port=5
  rotz [deg] : Outport  Port=6
  GPS lat [deg] : Outport  Port=7
  GPS long [deg] : Outport  Port=8
  GPS alt [m] : Outport  Port=9
  velocity [m/s] : Outport  Port=10
  heading [deg] : Outport  Port=11
  yaw rate [deg/s] : Outport  Port=12
  wires:
  Demux3/4 -> Gain1/1
  Gain1/1 -> yaw rate [deg/s]/1
  Demux3/3 -> velocity [m/s]/1
  compas converter/1(heading [deg]) -> heading [deg]/1
  xyz2GPS/1 -> Demux4/1
  Demux4/3 -> GPS alt [m]/1
  Demux4/2 -> GPS long [deg]/1
  Demux4/1 -> GPS lat [deg]/1
  Demux3/2 -> Gain/1, Selector/1
  Demux3/1 -> xyz2GPS/1, Demux1/1
  SELF/1 -> Demux3/1
  Demux2/3 -> rotz [deg]/1
  Demux2/2 -> roty [deg]/1
  Demux2/1 -> rotx [deg]/1
  Demux1/3 -> z [m]/1
  Demux1/2 -> y [m]/1
  Demux1/1 -> x [m]/1
  Gain/1 -> Demux2/1
  Selector/1 -> compas converter/1(rotz [rad])

== system Demo_DSRC_DNPW_cs/BMW_X5_1/Trajectories ==
  ElapsedTrack1 : Subsystem  Tag=ElapsedTrack  mask(PreScan Demux Block:){Filename='PathFollowerSva_2_Path.mat'}
      mask prompts: Filename "Name path-file"
      mask init:
      | route=load(['trajectories/',Filename]);
      | 
      | s=route.path(1,:);
      | x=route.path(2,:);
      | y=route.path(3,:);
      | z=route.path(4,:);
      | roll=route.path(5,:);
      | pitch=route.path(6,:);
      | yaw=route.path(7,:);
      settings: DeleteFcn=PreScanBlockDeleteFcn;
  Integrator1 : DiscreteIntegrator  Tag=TrajIntegrator  SampleTime=1/20  ICPrevOutput=DiscIntNeverNeededParam  ICPrevScaledInput=DiscIntNeverNeededParam
  PathFollowerSva_2 : Subsystem  Tag=Trajectory  mask(PreScan Source Block: Trajectory){FileName='PathFollowerSva_2_Synced.mat', TimeStep=1/20}
      mask prompts: TimeStep "Time Step [s]"
      mask help:
      | The Trajectory block contains the trajectories defined in the PreScan Experiment Editor. The output of the trajectory block is the (vehicle) State.
      |
      | For more information, please click Help.
      mask init:
      | [direc,name]=fileparts(get_param(bdroot, 'FileName'));
      | load([direc,'/Trajectories/',FileName])
      | trajectory=trajectory';
      | 
      | traj.time=trajectory(:,1);%[];
      | traj.signals.values=trajectory(:,2:19);
      | traj.dimensions=18;
      | traj.label='';
      | 
      | SampleTime=traj.time(2)-traj.time(1);
      settings: DeleteFcn=PreScanBlockDeleteFcn;
      mask Help: eval('openHelp(312)')
      mask Display: fprintf(FileName)
  PathFollowerSva_2_Offset : Constant  Tag=TrajectoryOffset  Value="[0  0  0  0  0  0]"
  Selector1 : Constant  Tag=TrajSubSelector  Value=2
  Traj2State1 : Subsystem  Tag=Traj2State
      settings: DeleteFcn=PreScanBlockDeleteFcn;
      mask Type: PreScan Demux Block:
  TrajSwitch1 : MultiPortSwitch  Tag=TrajSubSwitch  Inputs=2  zeroidx=off
  Velocity1 : Constant  Tag=TrajVelocity  Value=22.2222
  State : Outport  Tag=TrajOutport
  wires:
  PathFollowerSva_2/1(trajectory) -> Traj2State1/1(Traj Org)
  PathFollowerSva_2_Offset/1 -> Traj2State1/2(Offset), ElapsedTrack1/1(Offset)
  Integrator1/1 -> ElapsedTrack1/2(s)
  Velocity1/1 -> Integrator1/1
  Selector1/1 -> TrajSwitch1/1
  Traj2State1/1(state) -> TrajSwitch1/2
  ElapsedTrack1/1(state) -> TrajSwitch1/3
  TrajSwitch1/1 -> State/1

== system Demo_DSRC_DNPW_cs/BMW_X5_1/VISUSteer_Mux ==
  Column [deg] : Inport
  Steer [deg] : Inport  Port=2
  Mux2 : Mux  Inputs=2
  Steer : Outport
  wires:
  Column [deg]/1 -> Mux2/2
  Mux2/1 -> Steer/1
  Steer [deg]/1 -> Mux2/1

== system Demo_DSRC_DNPW_cs/CollisionDetection/retrieve CollisionDetection signal ==
  In : Inport
  Constant1 : Constant  Value=0
  Relational Operator : RelationalOperator  Operator=>  OutDataTypeStr=boolean
  Selector : Selector  InputPortWidth=10  IndexOptions=Index vector (dialog)  Indices=[1 3 5 7 9]  OutputSizes=1
  Out : Outport
  wires:
  Relational Operator/1 -> Out/1
  In/1 -> Selector/1
  Selector/1 -> Relational Operator/1
  Constant1/1 -> Relational Operator/2

== system Demo_DSRC_DNPW_cs/Fiat_Bravo_1/DSRC Transmitter ==
  Data : Inport
  Enable : EnablePort  PropagateVarSize=During execution
  DSRC_T_BusAssignment : BusAssignment  Tag=BusDSRCT  AssignedSignals=spare_1,spare_2,spare_3,spare_4,spare_5,spare_6,spare_7,spare_8,spare_9,spare_10,spare_11,spare_12,spare_13,spare_14,spare_15,spare_16,spare_17,spare_18,spare_19
  DSRC_T_Mux : Subsystem  Tag=MuxDSRCT
      settings: DeleteFcn=PreScanBlockDeleteFcn;
      mask Type: PreScan Mux Block:
      mask Display:
      | port_label('input', 1, 'Warning signal ID')
      | port_label('input', 2, 'Maneuvre ID')
      | port_label('input', 3, 'Vehicle Type')
      | port_label('input', 4, 'Braking Capacity')
      | port_label('input', 5, 'Vehicle Size')
      | port_label('input', 6, 'spare')
  Demux : Demux  Outputs=19
  Ground_{4..8} (5 alike) : Ground
  DSRC_T : Outport  Tag=AntennaTOutport
  wires:
  Demux/19 -> DSRC_T_BusAssignment/20  "Vehicle Height"
  Demux/18 -> DSRC_T_BusAssignment/19  "Vehicle Width"
  Demux/17 -> DSRC_T_BusAssignment/18  "Brakes"
  Demux/16 -> DSRC_T_BusAssignment/17  "Yaw rate"
  Demux/15 -> DSRC_T_BusAssignment/16  "Veritical Acc"
  Demux/14 -> DSRC_T_BusAssignment/15  "Lateral Acc"
  Demux/13 -> DSRC_T_BusAssignment/14  "Longitudinal Acc"
  Demux/12 -> DSRC_T_BusAssignment/13  "Angle"
  Demux/11 -> DSRC_T_BusAssignment/12  "Heading"
  Demux/10 -> DSRC_T_BusAssignment/11  "Speed"
  Demux/9 -> DSRC_T_BusAssignment/10  "Transmission State"
  Demux/8 -> DSRC_T_BusAssignment/9  "Accuracy"
  Demux/7 -> DSRC_T_BusAssignment/8  "Elevation"
  Demux/6 -> DSRC_T_BusAssignment/7  "Longitudinal"
  Demux/5 -> DSRC_T_BusAssignment/6  "Lateral"
  Ground_8/1 -> DSRC_T_Mux/5(vehicle_size)  "l50"
  Ground_7/1 -> DSRC_T_Mux/4(brakingcapacity)  "l49"
  Ground_6/1 -> DSRC_T_Mux/3(vehicle_type)  "l48"
  Ground_5/1 -> DSRC_T_Mux/2(maneuvre_id)  "l47"
  Ground_4/1 -> DSRC_T_Mux/1(warning_signal_id)  "l46"
  DSRC_T_Mux/1(Out1) -> DSRC_T/1  "l60"
  DSRC_T_BusAssignment/1 -> DSRC_T_Mux/6(spare)  "l58"
  Demux/4 -> DSRC_T_BusAssignment/5  "SecMark"
  Demux/3 -> DSRC_T_BusAssignment/4  "TempId"
  Demux/2 -> DSRC_T_BusAssignment/3  "MsgCount"
  Demux/1 -> DSRC_T_BusAssignment/2  "MsgId"
  Data/1 -> Demux/1
  DSRC_T_Mux/2(Out2) -> DSRC_T_BusAssignment/1  "L29"

== system Demo_DSRC_DNPW_cs/Fiat_Bravo_1/J2735 Encoder Basic Safety Message ==
  Msg : Inport
  Enable : EnablePort  PropagateVarSize=During execution
  Constant : Constant
  Demux : Demux  Outputs=19
  Embedded MATLAB Function : Stateflow chart  TreatAsAtomicUnit=on
  f() : Outport  InitialOutput=[1]
  Data : Outport  Port=2
  wires:
  Embedded MATLAB Function/1(y) -> Data/1
  Demux/19 -> Embedded MATLAB Function/19(u19)
  Demux/18 -> Embedded MATLAB Function/18(u18)
  Demux/17 -> Embedded MATLAB Function/17(u17)
  Demux/16 -> Embedded MATLAB Function/16(u16)
  Demux/15 -> Embedded MATLAB Function/15(u15)
  Demux/14 -> Embedded MATLAB Function/14(u14)
  Demux/13 -> Embedded MATLAB Function/13(u13)
  Demux/12 -> Embedded MATLAB Function/12(u12)
  Demux/11 -> Embedded MATLAB Function/11(u11)
  Demux/10 -> Embedded MATLAB Function/10(u10)
  Demux/9 -> Embedded MATLAB Function/9(u9)
  Demux/8 -> Embedded MATLAB Function/8(u8)
  Demux/7 -> Embedded MATLAB Function/7(u7)
  Demux/6 -> Embedded MATLAB Function/6(u6)
  Demux/5 -> Embedded MATLAB Function/5(u5)
  Demux/4 -> Embedded MATLAB Function/4(u4)
  Demux/3 -> Embedded MATLAB Function/3(u3)
  Demux/2 -> Embedded MATLAB Function/2(u2)
  Demux/1 -> Embedded MATLAB Function/1(u1)
  Constant/1 -> f()/1  "Enabled"
  Msg/1 -> Demux/1
